simulink model "ctnFCS"  (Simulink 8.1)
settings: Solver=ode45  StartTime=0.0  StopTime=10.0  RelTol=1e-3
values from neighbouring files (symbols this model uses):
  fcsParams = evalin('base', 'fcsParams')    [ctnNbParams.m]
libraries: NbLibrary x35
settings Model: Creator=sgras  LastModifiedBy=yamw
settings DataIOCC: SignalLoggingSaveFormat=Dataset
settings DebuggingCC: FcnCallInpInsideContextMsg=EnableAllAsError
settings GRTTargetCC: CodeReplacementLibrary=None  CombineOutputUpdateFcns=on  CPPClassGenCompliant=on  GRTInterface=off

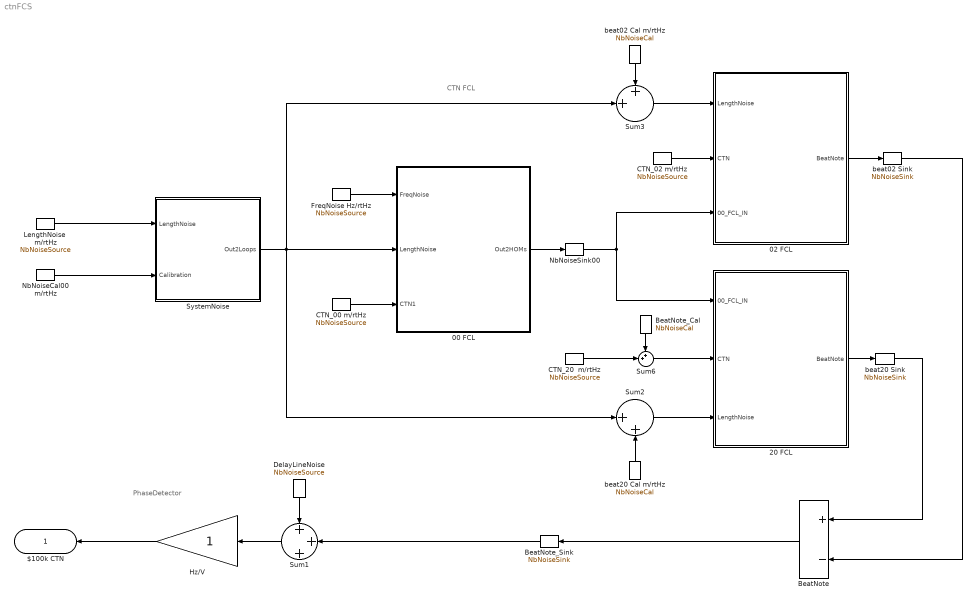
== system ctnFCS ==
  note: PhaseDetector
  note: CTN FCL
  00 FCL : Subsystem
  02 FCL : Subsystem
  20 FCL : Subsystem
  BeatNote : Sum  Inputs=+-
  BeatNote_Cal : NbLibrary/NbNoiseCal  Tag=NbNoiseCal  dof='BeatNote'  unit='m/rtHz'
      settings: AttributesFormatString=%<Tag>
  BeatNote_Sink : NbLibrary/NbNoiseSink  Tag=NbNoiseSink  dof='BeatNote'
      settings: AttributesFormatString=%<Tag>
  CTN_00 m/rtHz : NbLibrary/NbNoiseSource  Tag=NbNoiseSource  asd=fcsParams.ctnNb.CTN  groupNest=2  group='00 FCL'  subgroup='Coating'  subsubgroup=''  subsubsubgroup=''
      settings: AttributesFormatString=%<Tag>
  CTN_02 m/rtHz : NbLibrary/NbNoiseSource  Tag=NbNoiseSource  asd=fcsParams.ctnNb.CTN  groupNest=2  group='02 FCL'  subgroup='Coating'  subsubgroup=''  subsubsubgroup=''
      settings: AttributesFormatString=%<Tag>
  CTN_20  m/rtHz : NbLibrary/NbNoiseSource  Tag=NbNoiseSource  asd=fcsParams.ctnNb.CTN  groupNest=2  group='20 FCL'  subgroup='Coating'  subsubgroup=''  subsubsubgroup=''
      settings: AttributesFormatString=%<Tag>
  DelayLineNoise : NbLibrary/NbNoiseSource  Tag=NbNoiseSource  asd=0  groupNest=1  group=''  subgroup=''  subsubgroup=''  subsubsubgroup=''
      settings: AttributesFormatString=%<Tag>
  FreqNoise Hz/rtHz : NbLibrary/NbNoiseSource  Tag=NbNoiseSource  asd=fcsParams.ctnNb.LaserFreqNoise * (100 ./ fcsParams.freq)  groupNest=2  group='00 FCL'  subgroup='Freq'  subsubgroup=''  subsubsubgroup=''
      settings: AttributesFormatString=%<Tag>
  Hz/V : Gain
  LengthNoise  m/rtHz : NbLibrary/NbNoiseSource  Tag=NbNoiseSource  asd=fcsParams.ctnNb.noiseLength  groupNest=2  group='00 FCL'  subgroup='Length'  subsubgroup=''  subsubsubgroup=''
      settings: AttributesFormatString=%<Tag>
  NbNoiseCal00 m/rtHz : NbLibrary/NbNoiseCal  Tag=NbNoiseCal  dof='00'  unit='m/rtHz'
      settings: AttributesFormatString=%<Tag>
  NbNoiseSink00 : NbLibrary/NbNoiseSink  Tag=NbNoiseSink  dof='00'
      settings: AttributesFormatString=%<Tag>
  Sum1 : Sum  Inputs=+++
  Sum2 : Sum  Inputs=|++
  Sum3 : Sum  Inputs=++|
  Sum6 : Sum  Inputs=++|
  SystemNoise : Subsystem
  beat02 Cal m/rtHz : NbLibrary/NbNoiseCal  Tag=NbNoiseCal  dof='beat02'  unit='m/rtHz'
      settings: AttributesFormatString=%<Tag>
  beat02 Sink : NbLibrary/NbNoiseSink  Tag=NbNoiseSink  dof='beat02'
      settings: AttributesFormatString=%<Tag>
  beat20 Cal m/rtHz : NbLibrary/NbNoiseCal  Tag=NbNoiseCal  dof='beat20'  unit='m/rtHz'
      settings: AttributesFormatString=%<Tag>
  beat20 Sink : NbLibrary/NbNoiseSink  Tag=NbNoiseSink  dof='beat20'
      settings: AttributesFormatString=%<Tag>
  $100k CTN : Outport
  wires:
  NbNoiseCal00 m/rtHz/1 -> SystemNoise/2(Calibration)
  LengthNoise  m/rtHz/1 -> SystemNoise/1(LengthNoise)
  CTN_02 m/rtHz/1 -> 02 FCL/2(CTN)
  CTN_20  m/rtHz/1 -> Sum6/2
  00 FCL/1(Out2HOMs) -> NbNoiseSink00/1
  NbNoiseSink00/1 -> 02 FCL/3(00_FCL_IN), 20 FCL/1(00_FCL_IN)
  02 FCL/1(BeatNote) -> beat02 Sink/1
  beat02 Sink/1 -> BeatNote/2
  20 FCL/1(BeatNote) -> beat20 Sink/1
  Sum1/1 -> Hz/V/1
  Hz/V/1 -> $100k CTN/1
  BeatNote_Sink/1 -> Sum1/2
  DelayLineNoise/1 -> Sum1/1
  SystemNoise/1(Out2Loops) -> Sum2/1, 00 FCL/2(LengthNoise), Sum3/2
  Sum2/1 -> 20 FCL/3(LengthNoise)
  beat20 Cal m/rtHz/1 -> Sum2/2
  Sum3/1 -> 02 FCL/1(LengthNoise)
  beat02 Cal m/rtHz/1 -> Sum3/1
  BeatNote/1 -> BeatNote_Sink/1
  FreqNoise Hz/rtHz/1 -> 00 FCL/1(FreqNoise)
  beat20 Sink/1 -> BeatNote/1
  CTN_00 m/rtHz/1 -> 00 FCL/3(CTN1)
  Sum6/1 -> 20 FCL/2(CTN)
  BeatNote_Cal/1 -> Sum6/1

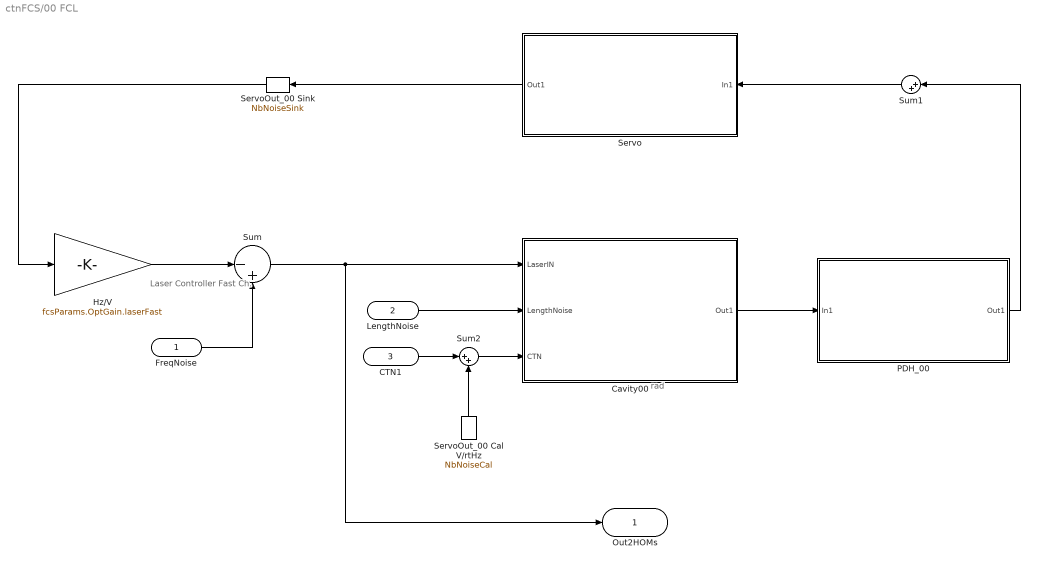
== system ctnFCS/00 FCL ==
  note: rad
  note: Laser Controller
      | Fast Ch.
  FreqNoise : Inport
  LengthNoise : Inport  Port=2
  CTN1 : Inport  Port=3
  Cavity00 : Subsystem
  Hz/V : Gain  Gain=fcsParams.OptGain.laserFast
  PDH_00 : Subsystem
  Servo : Subsystem
  ServoOut_00 Cal V/rtHz : NbLibrary/NbNoiseCal  Tag=NbNoiseCal  dof='ServoOut_00'  unit='V/rtHz'
      settings: AttributesFormatString=%<Tag>
  ServoOut_00 Sink : NbLibrary/NbNoiseSink  Tag=NbNoiseSink  dof='ServoOut_00'
      settings: AttributesFormatString=%<Tag>
  Sum : Sum  Inputs=|-+
  Sum1 : Sum  Inputs=|++
  Sum2 : Sum  Inputs=|++
  Out2HOMs : Outport
  wires:
  Cavity00/1(Out1) -> PDH_00/1(In1)
  Servo/1(Out1) -> ServoOut_00 Sink/1
  Hz/V/1 -> Sum/1
  FreqNoise/1 -> Sum/2
  LengthNoise/1 -> Cavity00/2(LengthNoise)
  CTN1/1 -> Sum2/1
  Sum/1 -> Cavity00/1(LaserIN), Out2HOMs/1
  Sum1/1 -> Servo/1(In1)
  PDH_00/1(Out1) -> Sum1/1
  ServoOut_00 Cal V/rtHz/1 -> Sum2/2
  ServoOut_00 Sink/1 -> Hz/V/1
  Sum2/1 -> Cavity00/3(CTN)

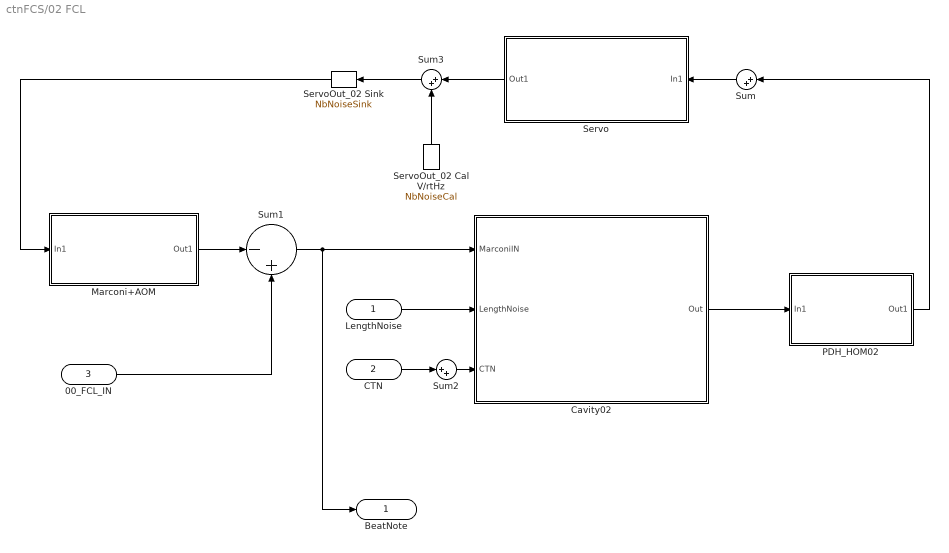
== system ctnFCS/02 FCL ==
  LengthNoise : Inport
  CTN : Inport  Port=2
  00_FCL_IN : Inport  Port=3
  Cavity02 : Subsystem
  Marconi+AOM : Subsystem
  PDH_HOM02 : Subsystem
  Servo : Subsystem
  ServoOut_02 Cal V/rtHz : NbLibrary/NbNoiseCal  Tag=NbNoiseCal  dof='ServoOut_02'  unit='V/rtHz'
      settings: AttributesFormatString=%<Tag>
  ServoOut_02 Sink : NbLibrary/NbNoiseSink  Tag=NbNoiseSink  dof='ServoOut_02'
      settings: AttributesFormatString=%<Tag>
  Sum : Sum  Inputs=|++
  Sum1 : Sum  Inputs=|-+
  Sum2 : Sum  Inputs=|++
  Sum3 : Sum  Inputs=|++
  BeatNote : Outport
  wires:
  Servo/1(Out1) -> Sum3/1
  Cavity02/1(Out) -> PDH_HOM02/1(In1)
  CTN/1 -> Sum2/1
  LengthNoise/1 -> Cavity02/2(LengthNoise)
  Sum/1 -> Servo/1(In1)
  PDH_HOM02/1(Out1) -> Sum/1
  Marconi+AOM/1(Out1) -> Sum1/1
  00_FCL_IN/1 -> Sum1/2
  Sum1/1 -> BeatNote/1, Cavity02/1(MarconiIN)
  Sum2/1 -> Cavity02/3(CTN)
  ServoOut_02 Sink/1 -> Marconi+AOM/1(In1)
  Sum3/1 -> ServoOut_02 Sink/1
  ServoOut_02 Cal V/rtHz/1 -> Sum3/2

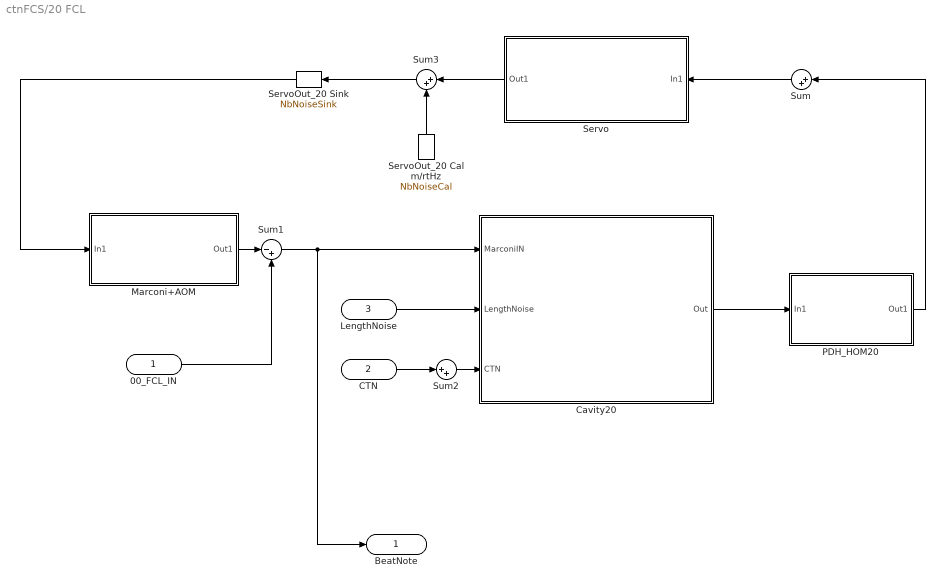
== system ctnFCS/20 FCL ==
  00_FCL_IN : Inport
  CTN : Inport  Port=2
  LengthNoise : Inport  Port=3
  Cavity20 : Subsystem
  Marconi+AOM : Subsystem
  PDH_HOM20 : Subsystem
  Servo : Subsystem
  ServoOut_20 Cal m/rtHz : NbLibrary/NbNoiseCal  Tag=NbNoiseCal  dof='ServoOut_20'  unit='m/rtHz'
      settings: AttributesFormatString=%<Tag>
  ServoOut_20 Sink : NbLibrary/NbNoiseSink  Tag=NbNoiseSink  dof='ServoOut_20'
      settings: AttributesFormatString=%<Tag>
  Sum : Sum  Inputs=|++
  Sum1 : Sum  Inputs=|-+
  Sum2 : Sum  Inputs=|++
  Sum3 : Sum  Inputs=|++
  BeatNote : Outport
  wires:
  Servo/1(Out1) -> Sum3/1
  Cavity20/1(Out) -> PDH_HOM20/1(In1)
  CTN/1 -> Sum2/1
  00_FCL_IN/1 -> Sum1/2
  LengthNoise/1 -> Cavity20/2(LengthNoise)
  Sum/1 -> Servo/1(In1)
  PDH_HOM20/1(Out1) -> Sum/1
  Sum1/1 -> BeatNote/1, Cavity20/1(MarconiIN)
  Marconi+AOM/1(Out1) -> Sum1/1
  ServoOut_20 Sink/1 -> Marconi+AOM/1(In1)
  Sum2/1 -> Cavity20/3(CTN)
  ServoOut_20 Cal m/rtHz/1 -> Sum3/2
  Sum3/1 -> ServoOut_20 Sink/1

== system ctnFCS/SystemNoise ==
  LengthNoise : Inport
  Calibration : Inport  Port=2
  Sum1 : Sum  Inputs=++|
  Out2Loops : Outport
  wires:
  LengthNoise/1 -> Sum1/2
  Sum1/1 -> Out2Loops/1
  Calibration/1 -> Sum1/1

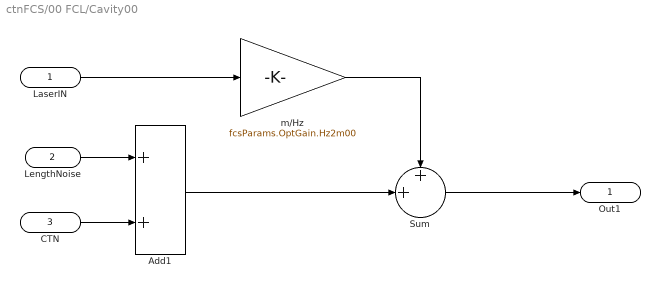
== system ctnFCS/00 FCL/Cavity00 ==
  LaserIN : Inport
  LengthNoise : Inport  Port=2
  CTN : Inport  Port=3
  Add1 : Sum
  Sum : Sum  Inputs=++|
  m/Hz : Gain  Gain=fcsParams.OptGain.Hz2m00
  Out1 : Outport
  wires:
  LengthNoise/1 -> Add1/1
  CTN/1 -> Add1/2
  Add1/1 -> Sum/2
  LaserIN/1 -> m/Hz/1
  Sum/1 -> Out1/1
  m/Hz/1 -> Sum/1

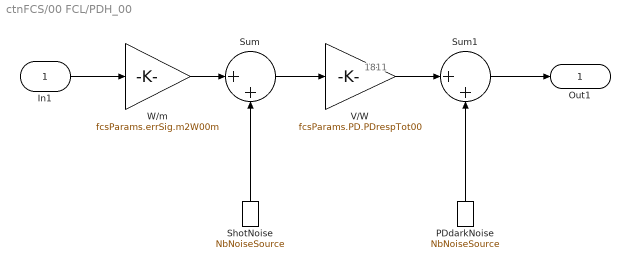
== system ctnFCS/00 FCL/PDH_00 ==
  note: 1811
  In1 : Inport
  " W/m" : Gain  Gain=fcsParams.errSig.m2W00m
  PDdarkNoise : NbLibrary/NbNoiseSource  Tag=NbNoiseSource  asd=fcsParams.ctnNb.n00PDOut  groupNest=2  group='00 FCL'  subgroup='PD'  subsubgroup=''  subsubsubgroup=''
      settings: AttributesFormatString=%<Tag>
  ShotNoise : NbLibrary/NbNoiseSource  Tag=NbNoiseSource  asd=fcsParams.ctnNb.PDshotNoise00  groupNest=2  group='00 FCL'  subgroup='Shot'  subsubgroup=''  subsubsubgroup=''
      settings: AttributesFormatString=%<Tag>
  Sum : Sum  Inputs=|++
  Sum1 : Sum  Inputs=|++
  V/W : Gain  Gain=fcsParams.PD.PDrespTot00
  Out1 : Outport
  wires:
  In1/1 -> " W/m"/1
  ShotNoise/1 -> Sum/2
  " W/m"/1 -> Sum/1
  Sum/1 -> V/W/1
  V/W/1 -> Sum1/1
  Sum1/1 -> Out1/1
  PDdarkNoise/1 -> Sum1/2

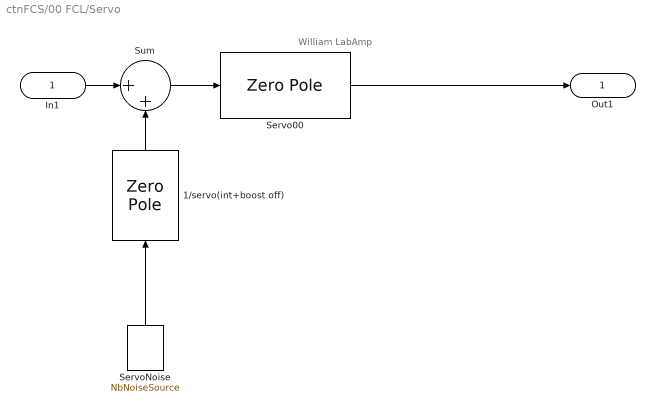
== system ctnFCS/00 FCL/Servo ==
  note: William LabAmp
  In1 : Inport
  1/servo(int+boost off) : ZeroPole  Zeros=2 * pi * fcsParams.servo00off.poles  Poles=2 * pi * fcsParams.servo00off.zeros  Gain=1/10^(fcsParams.servo00off.gain/20)
  Servo00 : ZeroPole  Zeros=-2*pi*fcsParams.servo00.zeros  Poles=-2 * pi *fcsParams.servo00.poles  Gain=10^(fcsParams.servo00.gain/20)
  ServoNoise : NbLibrary/NbNoiseSource  Tag=NbNoiseSource  asd=fcsParams.ctnNb.n00sServoOut  groupNest=2  group='00 FCL'  subgroup='Servo'  subsubgroup=''  subsubsubgroup=''
      settings: AttributesFormatString=%<Tag>
  Sum : Sum  Inputs=|++
  Out1 : Outport
  wires:
  Servo00/1 -> Out1/1
  Sum/1 -> Servo00/1
  In1/1 -> Sum/1
  ServoNoise/1 -> 1/servo(int+boost off)/1
  1/servo(int+boost off)/1 -> Sum/2

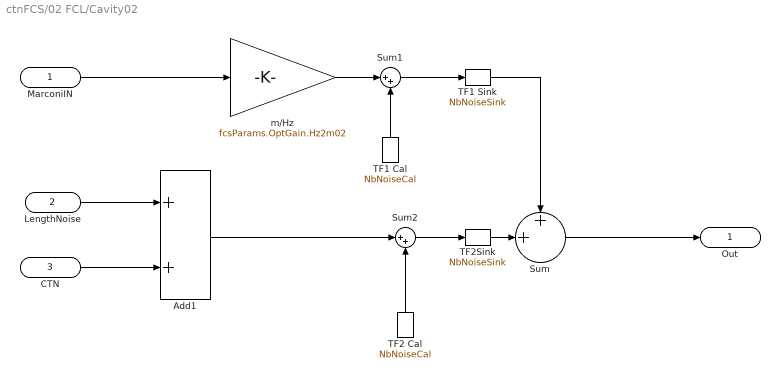
== system ctnFCS/02 FCL/Cavity02 ==
  MarconiIN : Inport
  LengthNoise : Inport  Port=2
  CTN : Inport  Port=3
  Add1 : Sum
  Sum : Sum  Inputs=++|
  Sum1 : Sum  Inputs=|++
  Sum2 : Sum  Inputs=|++
  TF1 Cal : NbLibrary/NbNoiseCal  Tag=NbNoiseCal  dof='TF1'  unit='rad/rad'
      settings: AttributesFormatString=%<Tag>
  "TF1 Sink " : NbLibrary/NbNoiseSink  Tag=NbNoiseSink  dof='TF1'
      settings: AttributesFormatString=%<Tag>
  "TF2 Cal " : NbLibrary/NbNoiseCal  Tag=NbNoiseCal  dof='TF2'  unit='rad/rad'
      settings: AttributesFormatString=%<Tag>
  TF2Sink : NbLibrary/NbNoiseSink  Tag=NbNoiseSink  dof='TF2'
      settings: AttributesFormatString=%<Tag>
  m/Hz : Gain  Gain=fcsParams.OptGain.Hz2m02
  Out : Outport
  wires:
  LengthNoise/1 -> Add1/1
  CTN/1 -> Add1/2
  Add1/1 -> Sum2/1
  Sum/1 -> Out/1
  m/Hz/1 -> Sum1/1
  MarconiIN/1 -> m/Hz/1
  Sum1/1 -> "TF1 Sink "/1
  Sum2/1 -> TF2Sink/1
  "TF1 Sink "/1 -> Sum/1
  TF2Sink/1 -> Sum/2
  TF1 Cal/1 -> Sum1/2
  "TF2 Cal "/1 -> Sum2/2

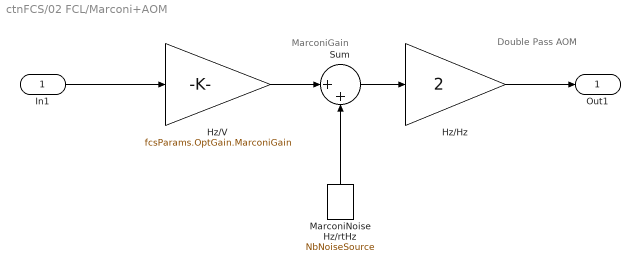
== system ctnFCS/02 FCL/Marconi+AOM ==
  note: MarconiGain
  note: Double Pass AOM
  In1 : Inport
  "Hz/Hz " : Gain  Gain=2
  Hz/V : Gain  Gain=fcsParams.OptGain.MarconiGain
  MarconiNoise Hz/rtHz : NbLibrary/NbNoiseSource  Tag=NbNoiseSource  asd=fcsParams.ctnNb.n02Marconi  groupNest=2  group='02 FCL'  subgroup='Marconi'  subsubgroup=''  subsubsubgroup=''
      settings: AttributesFormatString=%<Tag>
  Sum : Sum  Inputs=|++
  Out1 : Outport
  wires:
  MarconiNoise Hz/rtHz/1 -> Sum/2
  "Hz/Hz "/1 -> Out1/1
  Hz/V/1 -> Sum/1
  In1/1 -> Hz/V/1
  Sum/1 -> "Hz/Hz "/1

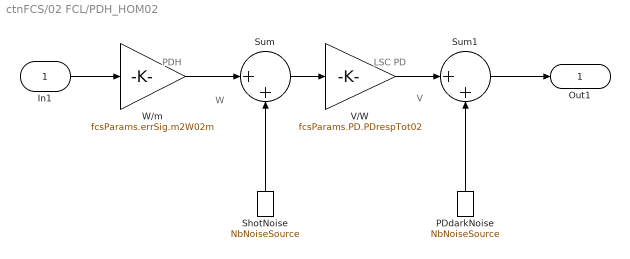
== system ctnFCS/02 FCL/PDH_HOM02 ==
  note: PDH
  note: W
  note: V
  note: LSC PD
  In1 : Inport
  " W/m" : Gain  Gain=fcsParams.errSig.m2W02m
  PDdarkNoise : NbLibrary/NbNoiseSource  Tag=NbNoiseSource  asd=fcsParams.ctnNb.n02PDOut  groupNest=2  group='02 FCL'  subgroup='PD'  subsubgroup=''  subsubsubgroup=''
      settings: AttributesFormatString=%<Tag>
  ShotNoise : NbLibrary/NbNoiseSource  Tag=NbNoiseSource  asd=fcsParams.ctnNb.PDshotNoise02  groupNest=2  group='02 FCL'  subgroup='Shot'  subsubgroup=''  subsubsubgroup=''
      settings: AttributesFormatString=%<Tag>
  Sum : Sum  Inputs=|++
  Sum1 : Sum  Inputs=|++
  V/W : Gain  Gain=fcsParams.PD.PDrespTot02
  Out1 : Outport
  wires:
  In1/1 -> " W/m"/1
  ShotNoise/1 -> Sum/2
  " W/m"/1 -> Sum/1
  Sum/1 -> V/W/1
  V/W/1 -> Sum1/1
  Sum1/1 -> Out1/1
  PDdarkNoise/1 -> Sum1/2

== system ctnFCS/02 FCL/Servo ==
  In1 : Inport
  Servo : ZeroPole  Zeros=-2 * pi * fcsParams.servo02.zeros  Poles=-2 * pi * fcsParams.servo02.poles  Gain=10^(fcsParams.servo02.gain/20)
  ServoNoise : NbLibrary/NbNoiseSource  Tag=NbNoiseSource  asd=fcsParams.ctnNb.n02sServoOut  groupNest=2  group='02 FCL'  subgroup='Servo'  subsubgroup=''  subsubsubgroup=''
      settings: AttributesFormatString=%<Tag>
  Sum : Sum  Inputs=|++
  Out1 : Outport
  wires:
  Servo/1 -> Sum/1
  Sum/1 -> Out1/1
  ServoNoise/1 -> Sum/2
  In1/1 -> Servo/1

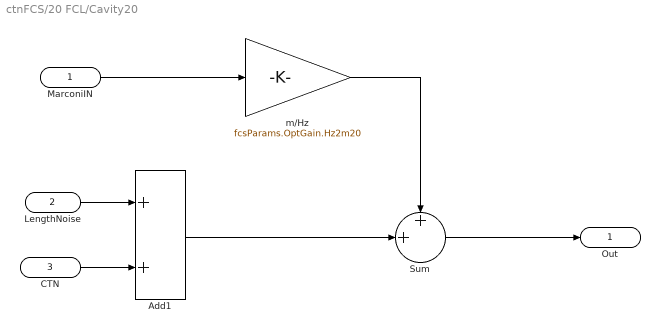
== system ctnFCS/20 FCL/Cavity20 ==
  MarconiIN : Inport
  LengthNoise : Inport  Port=2
  CTN : Inport  Port=3
  Add1 : Sum
  Sum : Sum  Inputs=++|
  m/Hz : Gain  Gain=fcsParams.OptGain.Hz2m20
  Out : Outport
  wires:
  LengthNoise/1 -> Add1/1
  CTN/1 -> Add1/2
  Add1/1 -> Sum/2
  Sum/1 -> Out/1
  m/Hz/1 -> Sum/1
  MarconiIN/1 -> m/Hz/1

== system ctnFCS/20 FCL/Marconi+AOM ==
  note: MarconiGain
  note: Double Pass AOM
  In1 : Inport
  "Hz/Hz " : Gain  Gain=2
  Hz/V : Gain  Gain=fcsParams.OptGain.MarconiGain
  MarconiNoise Hz/rtHz : NbLibrary/NbNoiseSource  Tag=NbNoiseSource  asd=fcsParams.ctnNb.n20Marconi  groupNest=2  group='20 FCL'  subgroup='Marconi'  subsubgroup=''  subsubsubgroup=''
      settings: AttributesFormatString=%<Tag>
  Sum : Sum  Inputs=|++
  Out1 : Outport
  wires:
  "Hz/Hz "/1 -> Out1/1
  Hz/V/1 -> Sum/1
  In1/1 -> Hz/V/1
  MarconiNoise Hz/rtHz/1 -> Sum/2
  Sum/1 -> "Hz/Hz "/1

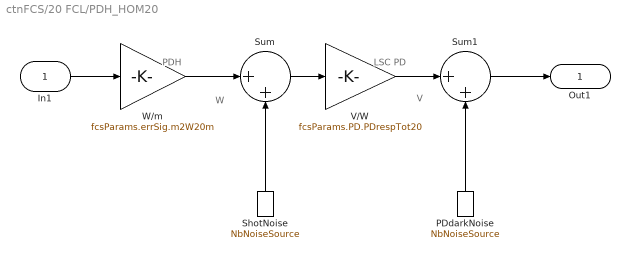
== system ctnFCS/20 FCL/PDH_HOM20 ==
  note: PDH
  note: W
  note: V
  note: LSC PD
  In1 : Inport
  " W/m" : Gain  Gain=fcsParams.errSig.m2W20m
  PDdarkNoise : NbLibrary/NbNoiseSource  Tag=NbNoiseSource  asd=fcsParams.ctnNb.n20PDOut  groupNest=2  group='20 FCL'  subgroup='PD'  subsubgroup=''  subsubsubgroup=''
      settings: AttributesFormatString=%<Tag>
  ShotNoise : NbLibrary/NbNoiseSource  Tag=NbNoiseSource  asd=fcsParams.ctnNb.PDshotNoise20  groupNest=2  group='20 FCL'  subgroup='Shot'  subsubgroup=''  subsubsubgroup=''
      settings: AttributesFormatString=%<Tag>
  Sum : Sum  Inputs=|++
  Sum1 : Sum  Inputs=|++
  V/W : Gain  Gain=fcsParams.PD.PDrespTot20
  Out1 : Outport
  wires:
  In1/1 -> " W/m"/1
  ShotNoise/1 -> Sum/2
  " W/m"/1 -> Sum/1
  Sum/1 -> V/W/1
  V/W/1 -> Sum1/1
  Sum1/1 -> Out1/1
  PDdarkNoise/1 -> Sum1/2

== system ctnFCS/20 FCL/Servo ==
  In1 : Inport
  Servo : ZeroPole  Zeros=-2 * pi * fcsParams.servo20.zeros  Poles=-2 * pi * fcsParams.servo20.poles  Gain=10^(fcsParams.servo20.gain/20)
  ServoNoise : NbLibrary/NbNoiseSource  Tag=NbNoiseSource  asd=fcsParams.ctnNb.n02sServoOut  groupNest=2  group='20 FCL'  subgroup='Servo'  subsubgroup=''  subsubsubgroup=''
      settings: AttributesFormatString=%<Tag>
  Sum : Sum  Inputs=|++
  Out1 : Outport
  wires:
  Servo/1 -> Sum/1
  Sum/1 -> Out1/1
  ServoNoise/1 -> Sum/2
  In1/1 -> Servo/1
